simulink model "final_project"  (R2017b)
settings: Solver=FixedStepAuto  StartTime=0.0  StopTime=stopTime  FixedStep=stepSize  RelTol=1e-3
InitFcn:
  | final_project_init
values from neighbouring files (symbols this model uses):
  carrierFreq = 5e6    (= 5000000)    [final_project_init.m]
  dataRate = 10e6    (= 10000000)    [final_project_init.m]
  detection_threshold = 100    [final_project_init.m]
  mapper_LUT_I = [1 0.70710678 0.70710678 0 -0.70710678 0 -1 -0.70710678]    [final_project_init.m]
  mapper_LUT_Q = [0 0.70710678 -0.70710678 -1 0.70710678 1 0 -0.70710678]    [final_project_init.m]
  memSize = 1024    [final_project_init.m]
  pilot_size = length(pilot_bits)    [final_project_init.m]
  sampleRate = clockRate    (= 40000000)    [final_project_init.m]
  stepSize = 1/sampleRate    (= 2.5e-08)    [final_project_init.m]
  symbolRate = dataRate/3    (= 3333333.33333)    [final_project_init.m]
  wordLength = 12    [final_project_init.m]
undefined symbols (not defined in the file or in its folder): AdvDSPBChannelOutDisplay, AdvDSPBDMemDisplay, dpoly, dspba, dspba_ChannelInVis, dspba_ChannelOutVis, dspba_internal_get_channel_ports, dspba_internal_get_demux_ports, evalAionMaskParam, latency, primtype, UseDontCare, value
libraries: DSPBAPrim x252, DSPBAControl x44, DSPBABase x32, DSPBAFilters x12, DSPBAVectorUtil x4
(part 1 of 4)
settings Model: Creator=bennetp  LastModifiedBy=soren
settings SolverCC: AutoInsertRateTranBlk=on

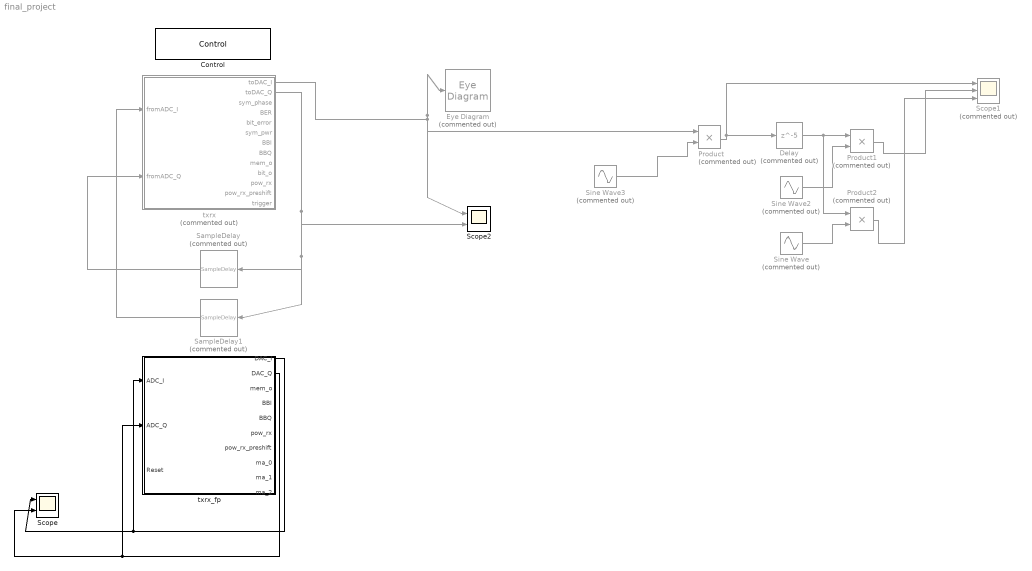
== system final_project ==
  Control : DSPBABase/Control  generate=off  language=VHDL  make_full_path=off  path_is_relative=on  autotestbench=on  signaldepth=2  coveragetestbench=off  logs=off  spacewidth=2  spacenum=1  addrwidth=10  datawidth=16  dataendian=Big Endian  hierarchicalnames=off  ramThresholdBits=-1  distRamThresholdBits=-1  mlabThresholdBits=-1  hardMultiplierThresholdLuts=-1  version=20150801  errorOnChanMismatch=1  errorOnGPIOMismatch=0  importModelsimResults=0  cycleAccurate=off  reinterpretCastMult=off  paramFile=final_project_params.xml
  Delay : Delay  Commented=on  DelayLength=5  InitialCondition=0  SampleTime=stepSize
  Eye Diagram : EyeDiagram  Commented=on
  Product : Product  Commented=on
  Product1 : Product  Commented=on
  Product2 : Product  Commented=on
  SampleDelay : DSPBAPrim/SampleDelay  Commented=on  primtype=sampdelay  nInputs=1  nOutputs=1  omode=Inherit via internal rule  otype=sfix(16)  scale=2^-15  rndmethod=Unbiased  factor=1  satmethod=Symmetric  shift_vec=[0 1 2 -1]  value=200  inPortNames=[' '; ' ';]  outPortNames=[' ']  dspbaimage=dspba_prim.jpg  text=dpoly(1, eye(1,value+1), 'z')  style=Optimised  visibilities=8 + 1024 + 2^17 + 2^18  flexible=off  slackgroup=0  augmented=0  version=20090407  advOptions=[]
  SampleDelay1 : DSPBAPrim/SampleDelay  Commented=on  primtype=sampdelay  nInputs=1  nOutputs=1  omode=Inherit via internal rule  otype=sfix(16)  scale=2^-15  rndmethod=Unbiased  factor=1  satmethod=Symmetric  shift_vec=[0 1 2 -1]  value=200  inPortNames=[' '; ' ';]  outPortNames=[' ']  dspbaimage=dspba_prim.jpg  text=dpoly(1, eye(1,value+1), 'z')  style=Optimised  visibilities=8 + 1024 + 2^17 + 2^18  flexible=off  slackgroup=0  augmented=0  version=20090407  advOptions=[]
  Scope : Scope  NumInputPorts=2
  Scope1 : Scope  Commented=on  NumInputPorts=3
  Scope2 : Scope  NumInputPorts=2
  Sine Wave : Sin  Commented=on  Frequency=carrierFreq*2*pi  Phase=pi  SampleTime=1/sampleRate
  Sine Wave2 : Sin  Commented=on  Frequency=carrierFreq*2*pi  Phase=pi/2  SampleTime=1/sampleRate
  Sine Wave3 : Sin  Commented=on  Frequency=carrierFreq*2*pi  Phase=pi/2  SampleTime=1/sampleRate
  txrx : Subsystem  Commented=on
  txrx_fp : Subsystem
  wires:
  Product1/1 -> Scope1/2
  Sine Wave2/1 -> Product1/2
  Product2/1 -> Scope1/3
  Sine Wave3/1 -> Product/2
  Delay/1 -> Product2/1, Product1/1
  txrx/2(toDAC_Q) -> SampleDelay1/1, SampleDelay/1, Scope2/2
  Product/1 -> Delay/1, Scope1/1
  Sine Wave/1 -> Product2/2
  txrx/1(toDAC_I) -> Eye Diagram/1, Product/1, Scope2/1
  SampleDelay/1 -> txrx/2(fromADC_Q)
  SampleDelay1/1 -> txrx/1(fromADC_I)
  txrx_fp/1(DAC_I) -> Scope/1, txrx_fp/1(ADC_I)
  txrx_fp/2(DAC_Q) -> Scope/2, txrx_fp/2(ADC_Q)

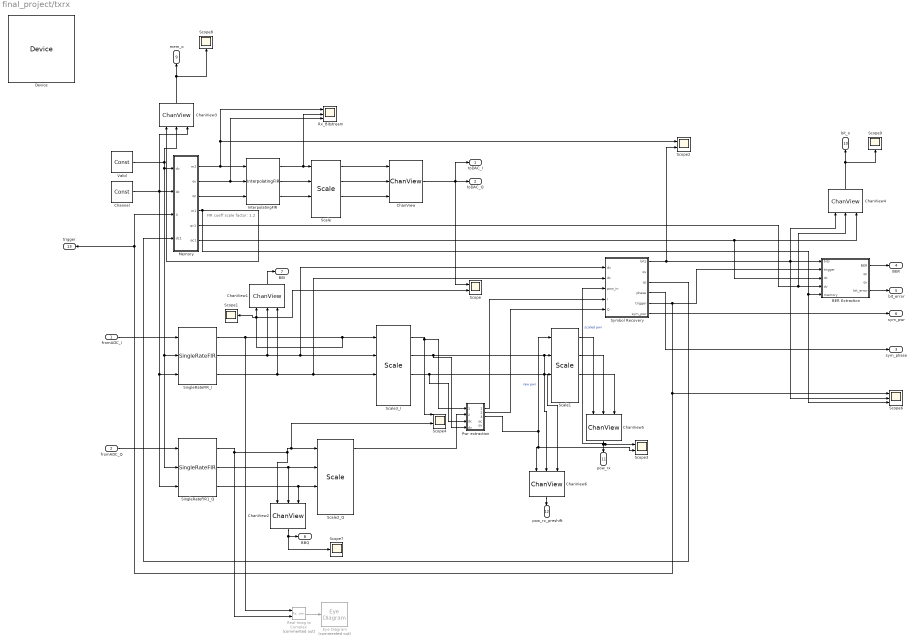
== system final_project/txrx ==
  note: FIR coeff scale factor: 1.2
  fromADC_I : Inport
  fromADC_Q : Inport  Port=2
  BER Extraction : Subsystem
  ChanView{,1..6} (7 alike) : DSPBABase/ChanView  nchans=1  chan_vector=[0]  outsvalid=off  latency=1  version=20090407
  Channel : DSPBAPrim/Const  primtype=const  nInputs=0  nOutputs=1  omode=Specify via dialog  otype=uint(8)  scale=1  rndmethod=Unbiased  factor=1  satmethod=Symmetric  shift_vec=[0 1 2 -1]  value=0  inPortNames=['+'; '+';]  outPortNames=[' ']  dspbaimage=dspba_prim.jpg  text=fprintf('%s', num2str(value));  style=Optimised  visibilities=8 + 1024  floatPrecision=float32_m23  version=20120820
  Device : DSPBABase/Device  family=Arria 10  stratix4device=Stratix IV E  hardcopy4device=HardCopy IV E  stratix5device=Stratix V GX  device=AUTO  speed=1  stratixSpeed=-5  stratix2Speed=-3  stratix3Speed=-2  stratix4gxSpeed=-2  stratix4gtSpeed=-1  cyclone2Speed=-6  cyclone3Speed=-7  arria2Speed=-4  cyclone4eSpeed=-8  stratix5Speed=-3  arria5Speed=-4  arriaSpeed=-6  cyclone3lsSpeed=-7  cyclone5Speed=-6  arria2gzSpeed=-3  nightFurySpeed=-2  ecp2Speed=-7  hardcopycompat=off  version=20140217  max10flashmode=off  max10nomeminit=off
  Eye Diagram : EyeDiagram  Commented=on
  InterpolatingFIR : DSPBAFilters/InterpolatingFIR  nInputRate=1  interp=sampleRate/dataRate  nchan=1  symmetry=Symmetrical  coef=fir.coeffs  addr=512  rwmode=Constant  nband=Use All Taps  exposebus=off  latency=8  version=20090407  recon=off  MM=[0,1,2,3,4,5,6,7,8,9,10,11,12,13,14,15]
  Memory : Subsystem
  Pwr extraction : Subsystem
  Real-Imag to Complex : RealImagToComplex  Commented=on
  Rx_Bitstream : Scope  NumInputPorts=3
  Scale : DSPBABase/Scale  otype=fixdt(1,12)  scale=1  rndmethod=Biased  factor=1  satmethod=Symmetric  shift_vec=13  latency=1  wideSimulation=off  version=20130807
  Scale1 : DSPBABase/Scale  otype=fixdt(1,wordLength)  scale=1  rndmethod=Biased  factor=1  satmethod=Symmetric  shift_vec=-11  latency=1  wideSimulation=off  version=20130807
  Scale2_Q : DSPBABase/Scale  otype=fixdt(1,wordLength)  scale=1  rndmethod=Biased  factor=1  satmethod=Symmetric  shift_vec=-3  latency=1  wideSimulation=off  version=20130807
  Scale3_I : DSPBABase/Scale  otype=fixdt(1,wordLength)  scale=1  rndmethod=Biased  factor=1  satmethod=Symmetric  shift_vec=-3  latency=1  wideSimulation=off  version=20130807
  Scope : Scope  NumInputPorts=2
  Scope{1,7..9} (4 alike) : Scope
  Scope2 : Scope  NumInputPorts=2
  Scope3 : Scope  NumInputPorts=2
  Scope4 : Scope  NumInputPorts=4
  Scope6 : Scope  NumInputPorts=3
  SingleRateFIR1_Q : DSPBAFilters/SingleRateFIR  nInputRate=40  nchan=1  symmetry=Symmetrical  coef=fir.coeffs  addr=512  rwmode=Read/Write  nband=Use All Taps  latency=4  exposebus=off  version=20090407  recon=off  MM=[0,1,2,3,4,5,6,7,8,9,10,11,12,13,14,15,16,17,18,19]
  SingleRateFIR_I : DSPBAFilters/SingleRateFIR  nInputRate=40  nchan=1  symmetry=Symmetrical  coef=fir.coeffs  addr=1024  rwmode=Read/Write  nband=Use All Taps  latency=4  exposebus=off  version=20090407  recon=off  MM=[0,1,2,3,4,5,6,7,8,9,10,11,12,13,14,15,16,17,18,19]
  Symbol Recovery : Subsystem
  Valid : DSPBAPrim/Const  primtype=const  nInputs=0  nOutputs=1  omode=boolean  otype=Boolean  scale=1  rndmethod=Unbiased  factor=1  satmethod=Symmetric  shift_vec=[0 1 2 -1]  value=1  inPortNames=['+'; '+';]  outPortNames=[' ']  dspbaimage=dspba_prim.jpg  text=fprintf('%s', num2str(value));  style=Optimised  visibilities=8 + 1024  floatPrecision=float32_m23  version=20120820
  toDAC_I : Outport
  toDAC_Q : Outport  Port=2
  sym_phase : Outport  Port=3
  BER : Outport  Port=4
  bit_error : Outport  Port=5
  sym_pwr : Outport  Port=6
  BBI : Outport  Port=7
  BBQ : Outport  Port=8
  mem_o : Outport  Port=9
  bit_o : Outport  Port=10
  pow_rx : Outport  Port=11
  pow_rx_preshift : Outport  Port=12
  trigger : Outport  Port=13
  wires:
  Valid/1 -> SingleRateFIR1_Q/2, SingleRateFIR_I/2, Memory/1(dv), ChanView3/2
  Channel/1 -> ChanView3/3, Memory/2(dc), SingleRateFIR1_Q/3, SingleRateFIR_I/3
  Memory/2(qv) -> Rx_Bitstream/3, InterpolatingFIR/2
  Memory/3(qc) -> InterpolatingFIR/3
  fromADC_I/1 -> SingleRateFIR_I/1
  fromADC_Q/1 -> SingleRateFIR1_Q/1
  Scale1/1 -> ChanView5/1
  Scale3_I/2 -> Pwr extraction/4(dv), ChanView6/2, Scale1/2
  Scale3_I/3 -> Pwr extraction/3(dc), ChanView6/3, Scale1/3
  ChanView/1 -> toDAC_I/1, toDAC_Q/1, Scope/1
  InterpolatingFIR/1 -> Rx_Bitstream/2, Scale/1
  InterpolatingFIR/2 -> Scale/2
  InterpolatingFIR/3 -> Scale/3
  Scale/1 -> ChanView/1
  Scale/2 -> ChanView/2
  Scale/3 -> ChanView/3
  Memory/1(m2) -> Scope2/1, Rx_Bitstream/1, InterpolatingFIR/1
  Symbol Recovery/1(bits) -> Scope2/2, BER Extraction/1(bits), ChanView4/1, Scope6/2
  Symbol Recovery/4(phase) -> sym_phase/1
  Memory/4(m1) -> ChanView3/1, Scope6/3, BER Extraction/5(memory)
  Memory/5(qv1) -> BER Extraction/4(dv), ChanView4/2
  Memory/6(qc1) -> BER Extraction/3(dc), ChanView4/3
  Symbol Recovery/5(trigger) -> Memory/3(trigger), trigger/1, Scope6/1, BER Extraction/2(trigger)
  Symbol Recovery/3(qc) -> Memory/4(dc1)
  BER Extraction/1(BER) -> BER/1
  BER Extraction/4(bit_error) -> bit_error/1
  Symbol Recovery/6(sym_pwr) -> sym_pwr/1
  SingleRateFIR1_Q/2 -> Scale2_Q/2, ChanView2/2
  SingleRateFIR1_Q/3 -> Scale2_Q/3, ChanView2/3
  SingleRateFIR_I/2 -> Scale3_I/2, Symbol Recovery/1(dv), ChanView1/2
  SingleRateFIR_I/3 -> Scale3_I/3, Symbol Recovery/2(dc), ChanView1/3
  Real-Imag to Complex/1 -> Eye Diagram/1
  ChanView2/1 -> Scope7/1, BBQ/1
  ChanView1/1 -> BBI/1
  ChanView3/1 -> mem_o/1, Scope8/1
  ChanView4/1 -> bit_o/1, Scope9/1
  Scale1/2 -> ChanView5/2
  Scale1/3 -> ChanView5/3
  ChanView5/1 -> pow_rx/1, Symbol Recovery/3(pow_in), Scope3/1  "scaled pwr"
  ChanView6/1 -> pow_rx_preshift/1
  SingleRateFIR1_Q/1 -> Scope4/3, Scale2_Q/1, ChanView2/1, Real-Imag to Complex/2
  SingleRateFIR_I/1 -> Scale3_I/1, Scope/2, Scope1/1, ChanView1/1, Real-Imag to Complex/1
  Pwr extraction/3(pwr) -> ChanView6/1, Scope3/2, Scale1/1  "raw pwr"
  Pwr extraction/1(Out1) -> Symbol Recovery/4(I)
  Pwr extraction/2(Out2) -> Symbol Recovery/5(Q)
  Scale2_Q/1 -> Pwr extraction/2(In2)
  Scale3_I/1 -> Pwr extraction/1(In1), Scope4/1

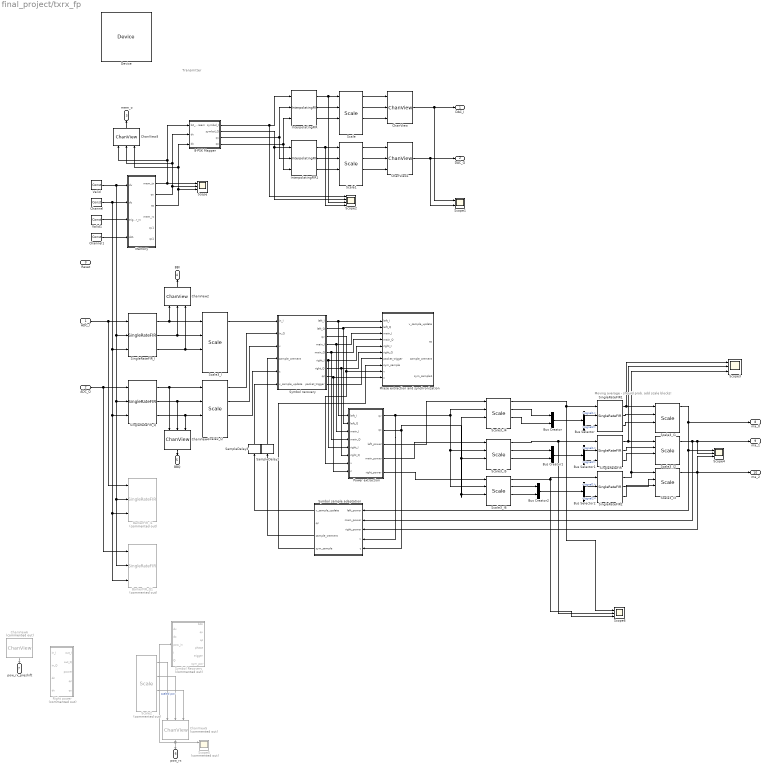
== system final_project/txrx_fp ==
  note: Moving average - should prob. add scale blocks!
  note: Transmitter
  ADC_I : Inport
  ADC_Q : Inport  Port=2
  Reset : Inport  Port=3
  8-PSK Mapper : Subsystem
  BarkerFIR_I1 : DSPBAFilters/SingleRateFIR  Commented=on  nInputRate=40  nchan=1  symmetry=Non Symmetrical  coef=barker_fir  addr=1024  rwmode=Read/Write  nband=Use All Taps  latency=2  exposebus=off  version=20090407  recon=off  MM=[0,1,2,3,4,5,6,7,8,9,10,11,12,13,14,15,16,17,18,19]
  BarkerFIR_Q1 : DSPBAFilters/SingleRateFIR  Commented=on  nInputRate=40  nchan=1  symmetry=Non Symmetrical  coef=barker_fir  addr=512  rwmode=Read/Write  nband=Use All Taps  latency=2  exposebus=off  version=20090407  recon=off  MM=[0,1,2,3,4,5,6,7,8,9,10,11,12,13,14,15,16,17,18,19]
  Bus Creator : BusCreator  Inputs=2
  Bus Creator1 : BusCreator  Inputs=2
  Bus Creator2 : BusCreator  Inputs=2
  Bus Selector : BusSelector  OutputSignals=signal1,signal2
  Bus Selector1 : BusSelector  OutputSignals=signal1,signal2
  Bus Selector2 : BusSelector  OutputSignals=signal1,signal2
  ChanView{,1..4} (5 alike) : DSPBABase/ChanView  nchans=1  chan_vector=[0]  outsvalid=off  latency=1  version=20090407
  ChanView5 : DSPBABase/ChanView  Commented=on  nchans=1  chan_vector=[0]  outsvalid=off  latency=1  version=20090407
  ChanView6 : DSPBABase/ChanView  Commented=on  nchans=1  chan_vector=[0]  outsvalid=off  latency=1  version=20090407
  Channel : DSPBAPrim/Const  primtype=const  nInputs=0  nOutputs=1  omode=Specify via dialog  otype=uint(8)  scale=1  rndmethod=Unbiased  factor=1  satmethod=Symmetric  shift_vec=[0 1 2 -1]  value=0  inPortNames=['+'; '+';]  outPortNames=[' ']  dspbaimage=dspba_prim.jpg  text=fprintf('%s', num2str(value));  style=Optimised  visibilities=8 + 1024  floatPrecision=float32_m23  version=20120820
  Channel1 : DSPBAPrim/Const  primtype=const  nInputs=0  nOutputs=1  omode=Specify via dialog  otype=uint(8)  scale=1  rndmethod=Unbiased  factor=1  satmethod=Symmetric  shift_vec=[0 1 2 -1]  value=0  inPortNames=['+'; '+';]  outPortNames=[' ']  dspbaimage=dspba_prim.jpg  text=fprintf('%s', num2str(value));  style=Optimised  visibilities=8 + 1024  floatPrecision=float32_m23  version=20120820
  Device : DSPBABase/Device  family=Arria 10  stratix4device=Stratix IV E  hardcopy4device=HardCopy IV E  stratix5device=Stratix V GX  device=AUTO  speed=1  stratixSpeed=-5  stratix2Speed=-3  stratix3Speed=-2  stratix4gxSpeed=-2  stratix4gtSpeed=-1  cyclone2Speed=-6  cyclone3Speed=-7  arria2Speed=-4  cyclone4eSpeed=-8  stratix5Speed=-3  arria5Speed=-4  arriaSpeed=-6  cyclone3lsSpeed=-7  cyclone5Speed=-6  arria2gzSpeed=-3  nightFurySpeed=-2  ecp2Speed=-7  hardcopycompat=off  version=20140217  max10flashmode=off  max10nomeminit=off
  InterpolatingFIR : DSPBAFilters/InterpolatingFIR  nInputRate=symbolRate/1e6  interp=3*sampleRate/dataRate  nchan=1  symmetry=Symmetrical  coef=fir.coeffs  addr=512  rwmode=Constant  nband=Use All Taps  exposebus=off  latency=8  version=20090407  recon=off  MM=[0,1,2,3,4,5,6,7,8,9,10,11,12,13,14,15]
  InterpolatingFIR1 : DSPBAFilters/InterpolatingFIR  nInputRate=symbolRate/1e6  interp=3*sampleRate/dataRate  nchan=1  symmetry=Symmetrical  coef=fir.coeffs  addr=512  rwmode=Constant  nband=Use All Taps  exposebus=off  latency=8  version=20090407  recon=off  MM=[0,1,2,3,4,5,6,7,8,9,10,11,12,13,14,15]
  Memory : Subsystem
  Phase extraction and synchronization : Subsystem
  Power extraction : Subsystem
  Right power : Subsystem  Commented=on
  SampleDelay1 : DSPBAPrim/SampleDelay  primtype=sampdelay  nInputs=1  nOutputs=1  omode=Inherit via internal rule  otype=sfix(16)  scale=2^-15  rndmethod=Unbiased  factor=1  satmethod=Symmetric  shift_vec=[0 1 2 -1]  value=1  inPortNames=[' '; ' ';]  outPortNames=[' ']  dspbaimage=dspba_prim.jpg  text=dpoly(1, eye(1,value+1), 'z')  style=Optimised  visibilities=8 + 1024 + 2^17 + 2^18  flexible=off  slackgroup=0  augmented=0  version=20090407  advOptions=[]
  SampleDelay3 : DSPBAPrim/SampleDelay  primtype=sampdelay  nInputs=1  nOutputs=1  omode=Inherit via internal rule  otype=sfix(16)  scale=2^-15  rndmethod=Unbiased  factor=1  satmethod=Symmetric  shift_vec=[0 1 2 -1]  value=1  inPortNames=[' '; ' ';]  outPortNames=[' ']  dspbaimage=dspba_prim.jpg  text=dpoly(1, eye(1,value+1), 'z')  style=Optimised  visibilities=8 + 1024 + 2^17 + 2^18  flexible=off  slackgroup=0  augmented=0  version=20090407  advOptions=[]
  Scale : DSPBABase/Scale  otype=fixdt(1,12)  scale=1  rndmethod=Biased  factor=1  satmethod=Symmetric  shift_vec=1  latency=1  wideSimulation=off  version=20130807
  Scale1 : DSPBABase/Scale  otype=fixdt(1,12)  scale=1  rndmethod=Biased  factor=1  satmethod=Symmetric  shift_vec=1  latency=1  wideSimulation=off  version=20130807
  Scale2 : DSPBABase/Scale  Commented=on  otype=fixdt(1,wordLength)  scale=1  rndmethod=Biased  factor=1  satmethod=Symmetric  shift_vec=-11  latency=1  wideSimulation=off  version=20130807
  Scale2_Q : DSPBABase/Scale  otype=fixdt(1,wordLength)  scale=1  rndmethod=Biased  factor=1  satmethod=Symmetric  shift_vec=-2  latency=1  wideSimulation=off  version=20130807
  Scale3_I : DSPBABase/Scale  otype=fixdt(1,wordLength)  scale=1  rndmethod=Biased  factor=1  satmethod=Symmetric  shift_vec=-2  latency=1  wideSimulation=off  version=20130807
  Scale3_I1 : DSPBABase/Scale  otype=fixdt(1,wordLength)  scale=1  rndmethod=Biased  factor=1  satmethod=Symmetric  shift_vec=-3  latency=1  wideSimulation=off  version=20130807
  Scale3_I2 : DSPBABase/Scale  otype=fixdt(1,wordLength)  scale=1  rndmethod=Biased  factor=1  satmethod=Symmetric  shift_vec=-3  latency=1  wideSimulation=off  version=20130807
  Scale3_I3 : DSPBABase/Scale  otype=fixdt(1,wordLength)  scale=1  rndmethod=Biased  factor=1  satmethod=Symmetric  shift_vec=-3  latency=1  wideSimulation=off  version=20130807
  Scale3_I4 : DSPBABase/Scale  otype=fixdt(1,18)  scale=1  rndmethod=Biased  factor=1  satmethod=Symmetric  shift_vec=-7  latency=1  wideSimulation=off  version=20130807
  Scale3_I5 : DSPBABase/Scale  otype=fixdt(1,18)  scale=1  rndmethod=Biased  factor=1  satmethod=Symmetric  shift_vec=-7  latency=1  wideSimulation=off  version=20130807
  Scale3_I6 : DSPBABase/Scale  otype=fixdt(1,18)  scale=1  rndmethod=Biased  factor=1  satmethod=Symmetric  shift_vec=-7  latency=1  wideSimulation=off  version=20130807
  Scope{,3..4,6} (4 alike) : Scope  NumInputPorts=3
  Scope1 : Scope  NumInputPorts=2
  Scope2 : Scope  NumInputPorts=4
  Scope5 : Scope  Commented=on  NumInputPorts=2
  SingleRateFIR : DSPBAFilters/SingleRateFIR  nInputRate=40  nchan=1  symmetry=Symmetrical  coef=moving_avg_fir  addr=2048  rwmode=Constant  nband=Use All Taps  latency=2  exposebus=off  version=20090407  recon=off  MM=[0,1,2,3,4,5,6,7,8,9,10,11,12,13,14,15,16,17,18,19]
  SingleRateFIR1 : DSPBAFilters/SingleRateFIR  nInputRate=40  nchan=1  symmetry=Symmetrical  coef=moving_avg_fir  addr=2048  rwmode=Constant  nband=Use All Taps  latency=2  exposebus=off  version=20090407  recon=off  MM=[0,1,2,3,4,5,6,7,8,9,10,11,12,13,14,15,16,17,18,19]
  SingleRateFIR2 : DSPBAFilters/SingleRateFIR  nInputRate=40  nchan=1  symmetry=Symmetrical  coef=moving_avg_fir  addr=2048  rwmode=Constant  nband=Use All Taps  latency=2  exposebus=off  version=20090407  recon=off  MM=[0,1,2,3,4,5,6,7,8,9,10,11,12,13,14,15,16,17,18,19]
  SingleRateFIR_I : DSPBAFilters/SingleRateFIR  nInputRate=40  nchan=1  symmetry=Symmetrical  coef=fir.coeffs  addr=1024  rwmode=Read/Write  nband=Use All Taps  latency=2  exposebus=off  version=20090407  recon=off  MM=[0,1,2,3,4,5,6,7,8,9,10,11,12,13,14,15,16,17,18,19]
  SingleRateFIR_Q : DSPBAFilters/SingleRateFIR  nInputRate=40  nchan=1  symmetry=Symmetrical  coef=fir.coeffs  addr=512  rwmode=Read/Write  nband=Use All Taps  latency=2  exposebus=off  version=20090407  recon=off  MM=[0,1,2,3,4,5,6,7,8,9,10,11,12,13,14,15,16,17,18,19]
  Symbol Recovery : Subsystem  Commented=on
  Symbol recovery : Subsystem
  Symbol sample adaptation : Subsystem
  Valid : DSPBAPrim/Const  primtype=const  nInputs=0  nOutputs=1  omode=boolean  otype=Boolean  scale=1  rndmethod=Unbiased  factor=1  satmethod=Symmetric  shift_vec=[0 1 2 -1]  value=1  inPortNames=['+'; '+';]  outPortNames=[' ']  dspbaimage=dspba_prim.jpg  text=fprintf('%s', num2str(value));  style=Optimised  visibilities=8 + 1024  floatPrecision=float32_m23  version=20120820
  Valid1 : DSPBAPrim/Const  primtype=const  nInputs=0  nOutputs=1  omode=boolean  otype=Boolean  scale=1  rndmethod=Unbiased  factor=1  satmethod=Symmetric  shift_vec=[0 1 2 -1]  value=0  inPortNames=['+'; '+';]  outPortNames=[' ']  dspbaimage=dspba_prim.jpg  text=fprintf('%s', num2str(value));  style=Optimised  visibilities=8 + 1024  floatPrecision=float32_m23  version=20120820
  DAC_I : Outport
  DAC_Q : Outport  Port=2
  mem_o : Outport  Port=3
  BBI : Outport  Port=4
  BBQ : Outport  Port=5
  pow_rx : Outport  Port=6
  pow_rx_preshift : Outport  Port=7
  ma_0 : Outport  Port=8
  ma_1 : Outport  Port=9
  ma_2 : Outport  Port=10
  wires:
  Valid/1 -> Memory/1(dv), SingleRateFIR_I/2, BarkerFIR_Q1/2, BarkerFIR_I1/2, SingleRateFIR_Q/2
  Channel/1 -> Memory/2(dc), SingleRateFIR_I/3, BarkerFIR_Q1/3, BarkerFIR_I1/3, SingleRateFIR_Q/3
  Memory/1(mem_tx) -> ChanView3/1, 8-PSK Mapper/1(bit_stream), Scope/1
  8-PSK Mapper/1(symbol_I) -> InterpolatingFIR/1, Scope2/1
  8-PSK Mapper/2(symbol_Q) -> Scope2/2, InterpolatingFIR1/1
  ChanView3/1 -> mem_o/1
  Memory/2(qv) -> ChanView3/2, 8-PSK Mapper/2(dv), Scope/2
  Memory/3(qc) -> ChanView3/3, 8-PSK Mapper/3(dc), Scope/3
  InterpolatingFIR/1 -> Scale/1, Scope2/3
  InterpolatingFIR1/1 -> Scope2/4, Scale1/1
  Scale/1 -> ChanView/1
  Scale1/1 -> ChanView1/1
  InterpolatingFIR1/2 -> Scale1/2
  InterpolatingFIR1/3 -> Scale1/3
  Scale1/3 -> ChanView1/3
  Scale1/2 -> ChanView1/2
  Scale/2 -> ChanView/2
  Scale/3 -> ChanView/3
  InterpolatingFIR/2 -> Scale/2
  InterpolatingFIR/3 -> Scale/3
  ChanView/1 -> DAC_I/1, Scope1/1
  ChanView1/1 -> DAC_Q/1, Scope1/2
  8-PSK Mapper/3(qv) -> InterpolatingFIR/2, InterpolatingFIR1/2
  8-PSK Mapper/4(qc) -> InterpolatingFIR1/3, InterpolatingFIR/3
  ChanView5/1 -> Scope5/1, Symbol Recovery/3(pow_in), pow_rx/1  "scaled pwr"
  Scale2/2 -> ChanView5/2
  ChanView2/1 -> BBI/1
  Scale2/1 -> ChanView5/1
  Scale2/3 -> ChanView5/3
  ChanView4/1 -> BBQ/1
  ChanView6/1 -> pow_rx_preshift/1
  ADC_I/1 -> BarkerFIR_I1/1, SingleRateFIR_I/1
  ADC_Q/1 -> BarkerFIR_Q1/1, SingleRateFIR_Q/1
  SingleRateFIR_I/1 -> ChanView2/1, Scale3_I/1
  SingleRateFIR_I/2 -> Scale3_I/2, ChanView2/2
  SingleRateFIR_I/3 -> Scale3_I/3, ChanView2/3
  SingleRateFIR_Q/3 -> Scale2_Q/3, ChanView4/3
  SingleRateFIR_Q/2 -> Scale2_Q/2, ChanView4/2
  SingleRateFIR_Q/1 -> Scale2_Q/1, ChanView4/1
  Scale3_I/1 -> Symbol recovery/1(in_I)
  Scale2_Q/1 -> Symbol recovery/2(in_Q)
  Scale2_Q/2 -> Symbol recovery/3(v)
  Scale2_Q/3 -> Symbol recovery/5(c)
  Symbol recovery/1(left_I) -> Power extraction/1(left_I), Phase extraction and synchronization/1(left_I)
  Symbol recovery/2(left_Q) -> Power extraction/2(left_Q), Phase extraction and synchronization/2(left_Q)
  Symbol recovery/3(qv) -> Power extraction/7(v), Phase extraction and synchronization/9(v)
  Symbol recovery/4(main_I) -> Power extraction/3(main_I), Phase extraction and synchronization/3(main_I)
  Symbol recovery/5(main_Q) -> Phase extraction and synchronization/4(main_Q), Power extraction/4(main_Q)
  Symbol recovery/7(right_Q) -> Power extraction/6(right_Q), Phase extraction and synchronization/6(right_Q)
  Symbol recovery/8(qc) -> Power extraction/8(c), Phase extraction and synchronization/10(c)
  Symbol sample adaptation/3(sample_crement) -> SampleDelay1/1
  Power extraction/2(qc) -> Symbol sample adaptation/5(c), Scale3_I5/3, Scale3_I4/3, Scale3_I6/3
  Power extraction/1(qv) -> Symbol sample adaptation/4(v), Scale3_I6/2, Scale3_I5/2, Scale3_I4/2
  SingleRateFIR1/1 -> Scale3_I1/1, Scope3/1
  SingleRateFIR/1 -> Scale3_I2/1, Scope3/2
  SingleRateFIR2/1 -> Scale3_I3/1, Scope3/3
  Symbol sample adaptation/1(v_sample_update) -> SampleDelay3/1
  SampleDelay3/1 -> Symbol recovery/6(v_sample_update)
  SampleDelay1/1 -> Symbol recovery/4(sample_crement)
  Symbol recovery/9(packet_trigger) -> Phase extraction and synchronization/7(packet_trigger)
  Symbol sample adaptation/4(sym_sample) -> Phase extraction and synchronization/8(sym_sample)
  Symbol recovery/6(right_I) -> Phase extraction and synchronization/5(right_I), Power extraction/5(right_I)
  SingleRateFIR1/2 -> Scale3_I1/2
  SingleRateFIR1/3 -> Scale3_I1/3
  SingleRateFIR/2 -> Scale3_I2/2
  SingleRateFIR/3 -> Scale3_I2/3
  SingleRateFIR2/2 -> Scale3_I3/2
  SingleRateFIR2/3 -> Scale3_I3/3
  Scale3_I1/1 -> ma_0/1, Symbol sample adaptation/1(left_power), Scope4/1
  Scale3_I2/1 -> Symbol sample adaptation/2(main_power), ma_1/1, Scope4/2
  Channel1/1 -> Memory/4(dc1)
  Valid1/1 -> Memory/3(trigger_rx)
  Scale3_I3/1 -> ma_2/1, Symbol sample adaptation/3(right_power), Scope4/3
  Power extraction/3(left_power) -> Scale3_I4/1
  Power extraction/4(main_power) -> Scale3_I5/1
  Power extraction/5(right_power) -> Scale3_I6/1
  Scale3_I4/1 -> Scope6/1, SingleRateFIR1/1
  Scale3_I5/1 -> Scope6/2, SingleRateFIR/1
  Scale3_I6/1 -> SingleRateFIR2/1, Scope6/3
  Scale3_I4/2 -> Bus Creator/1
  Scale3_I4/3 -> Bus Creator/2
  Scale3_I5/2 -> Bus Creator1/1
  Scale3_I5/3 -> Bus Creator1/2
  Scale3_I6/2 -> Bus Creator2/1
  Scale3_I6/3 -> Bus Creator2/2
  Bus Creator/1 -> Bus Selector/1
  Bus Selector/1 -> SingleRateFIR1/2  "<signal1>"
  Bus Selector/2 -> SingleRateFIR1/3  "<signal2>"
  Bus Selector1/1 -> SingleRateFIR/2  "<signal1>"
  Bus Selector1/2 -> SingleRateFIR/3  "<signal2>"
  Bus Selector2/1 -> SingleRateFIR2/2  "<signal1>"
  Bus Selector2/2 -> SingleRateFIR2/3  "<signal2>"
  Bus Creator1/1 -> Bus Selector1/1
  Bus Creator2/1 -> Bus Selector2/1

== system final_project/txrx/BER Extraction ==
  note: BER Computation
  bits : Inport
  trigger : Inport  Port=2
  dc : Inport  Port=3
  dv : Inport  Port=4
  memory : Inport  Port=5
  And : DSPBAPrim/And  primtype=and  nInputs=2  nOutputs=1  omode=Inherit via internal rule  otype=sfix(16)  scale=2^-15  rndmethod=Unbiased  factor=1  satmethod=Symmetric  shift_vec=[0 1 2 -1]  value=0  inPortNames=[' '; ' '; ' '; ' '; ' '; ' '; ' '; ' '; ' '; ' '; ' '; ' '; ' '; ' '; ' '; ' '; ]  outPortNames=[' ']  dspbaimage=dspba_prim.jpg  text=fprintf('&');  style=Optimised  visibilities=8+2  version=20090407
  Bit counter : DSPBAPrim/Counter  Commented=on  primtype=counter  nInputs=1  nOutputs=1  omode=Inherit via internal rule  otype=ufix(16)  scale=2^-0  rndmethod=Unbiased  factor=1  satmethod=Symmetric  shift_vec=[0 1 2 -1]  value=[0 memSize 1]  inPortNames=[' '; ' ';]  outPortNames=[' ']  dspbaimage=dspba_prim.jpg  text=fprintf('counter\n[%d %d %d]', value(1), value(2), value(3));  style=Optimised  visibilities=8 + 1024  version=20090407
  ChannelIn : DSPBAPrim/ChannelIn  primtype=channelin  nInputs=dspba_internal_get_channel_ports(gcb)  nOutputs=dspba_internal_get_channel_ports(gcb)  omode=Inherit via internal rule  otype=sfix(16)  scale=2^-15  rndmethod=Unbiased  factor=1  satmethod=Symmetric  shift_vec=[0 1 2 -1]  value=3  inPortNames=['v'; 'c'; '0'; '1'; '2'; '3'; '4'; '5'; '6'; '7'; '8'; '9'; 'A'; 'B'; 'D'; 'E'; 'F'; 'G'; 'H'; 'I'; 'J'; 'K'; 'L'; 'M'; 'N'; 'O'; 'P'; 'Q'; 'R'; 'S'; 'T'; 'U'; 'W'; 'X'; 'Y'; 'Z']  outPortNames=['v'; 'c'; '0'; '1'; '2'; '3'; '4'; '5'; '6'; '7'; '8'; '9'; 'A'; 'B'; 'D'; 'E'; 'F'; 'G'; 'H'; 'I'; 'J'; 'K'; 'L'; 'M'; 'N'; 'O'; 'P'; 'Q'; 'R'; 'S'; 'T'; 'U'; 'W'; 'X'; 'Y'; 'Z']  dspbaimage=dspba_prim.jpg  text=fprintf('In');  style=Optimised  dataSignals=3  foldingEnabled=off  channels=1  sampleRate=200  packetBeginPresent=off  packetBeginEnabled=off  visibilities=dspba_ChannelInVis(gcb)  latencyCorrection=0  scheduleOrigin=on  version=20141013
  ChannelOut : DSPBAPrim/ChannelOut  primtype=channelout  nInputs=dspba_internal_get_channel_ports(gcb)  nOutputs=dspba_internal_get_channel_ports(gcb)  omode=Inherit via internal rule  otype=sfix(16)  scale=2^-15  rndmethod=Unbiased  factor=1  satmethod=Symmetric  shift_vec=[0 1 2 -1]  value=2  inPortNames=['v'; 'c'; '0'; '1'; '2'; '3'; '4'; '5'; '6'; '7'; '8'; '9'; 'A'; 'B'; 'D'; 'E'; 'F'; 'G'; 'H'; 'I'; 'J'; 'K'; 'L'; 'M'; 'N'; 'O'; 'P'; 'Q'; 'R'; 'S'; 'T'; 'U'; 'W'; 'X'; 'Y'; 'Z']  outPortNames=['v'; 'c'; '0'; '1'; '2'; '3'; '4'; '5'; '6'; '7'; '8'; '9'; 'A'; 'B'; 'D'; 'E'; 'F'; 'G'; 'H'; 'I'; 'J'; 'K'; 'L'; 'M'; 'N'; 'O'; 'P'; 'Q'; 'R'; 'S'; 'T'; 'U'; 'W'; 'X'; 'Y'; 'Z']  dspbaimage=dspba_prim.jpg  text=fprintf('Out%s', AdvDSPBChannelOutDisplay(latency));  style=Optimised  dataSignals=2  foldingEnabled=off  channels=1  sampleRate=200  packetBeginPresent=off  packetBeginEnabled=off  visibilities=dspba_ChannelOutVis(gcb)  latency=0  latencyCorrection=0  version=20141013
  CmpEQ : DSPBAPrim/CmpEQ  Commented=on  primtype=cmpeq  nInputs=2  nOutputs=1  omode=boolean  otype=sfix(16)  scale=2^-15  rndmethod=Unbiased  factor=1  satmethod=Symmetric  shift_vec=[0 1 2 -1]  value=0  inPortNames=[' '; ' ';]  outPortNames=[' ']  dspbaimage=dspba_prim.jpg  text=fprintf('==');  style=Optimised  visibilities=0  advOptions=[]  version=20130117
  CmpNE : DSPBAPrim/CmpNE  primtype=cmpne  nInputs=2  nOutputs=1  omode=boolean  otype=sfix(16)  scale=2^-15  rndmethod=Unbiased  factor=1  satmethod=Symmetric  shift_vec=[0 1 2 -1]  value=0  inPortNames=[' '; ' ';]  outPortNames=[' ']  dspbaimage=dspba_prim.jpg  text=fprintf('~=');  style=Optimised  visibilities=0  advOptions=[]  version=20130117
  Const : DSPBAPrim/Const  Commented=on  primtype=const  nInputs=0  nOutputs=1  omode=Inherit via internal rule  otype=sfix(16)  scale=2^-15  rndmethod=Unbiased  factor=1  satmethod=Symmetric  shift_vec=[0 1 2 -1]  value=0  inPortNames=['+'; '+';]  outPortNames=[' ']  dspbaimage=dspba_prim.jpg  text=fprintf('%s', num2str(value));  style=Optimised  visibilities=8 + 1024  floatPrecision=float32_m23  version=20120820
  Const1 : DSPBAPrim/Const  primtype=const  nInputs=0  nOutputs=1  omode=Inherit via internal rule  otype=sfix(16)  scale=2^-15  rndmethod=Unbiased  factor=1  satmethod=Symmetric  shift_vec=[0 1 2 -1]  value=0  inPortNames=['+'; '+';]  outPortNames=[' ']  dspbaimage=dspba_prim.jpg  text=fprintf('%s', num2str(value));  style=Optimised  visibilities=8 + 1024  floatPrecision=float32_m23  version=20120820
  Divide : DSPBAPrim/Divide  Commented=on  primtype=divide  nInputs=2  nOutputs=1  omode=Inherit via internal rule  otype=sfix(16)  scale=2^-15  rndmethod=Unbiased  factor=1  satmethod=Symmetric  shift_vec=[0 1 2 -1]  value=round([0:255]/17)  inPortNames=[' '; ' ';]  outPortNames=[' ']  dspbaimage=dspba_prim.jpg  text=fprintf('a\n----\nb');  style=Optimised  visibilities=8+2^17+2^18  floatRounding=correct  advOptions=[]  version=20130115
  Error counter : DSPBAPrim/Counter  Commented=on  primtype=counter  nInputs=1  nOutputs=1  omode=Inherit via internal rule  otype=ufix(16)  scale=2^-0  rndmethod=Unbiased  factor=1  satmethod=Symmetric  shift_vec=[0 1 2 -1]  value=[0 memSize 1]  inPortNames=[' '; ' ';]  outPortNames=[' ']  dspbaimage=dspba_prim.jpg  text=fprintf('counter\n[%d %d %d]', value(1), value(2), value(3));  style=Optimised  visibilities=8 + 1024  version=20090407
  Or : DSPBAPrim/Or  Commented=on  primtype=or  nInputs=2  nOutputs=1  omode=Inherit via internal rule  otype=sfix(16)  scale=2^-15  rndmethod=Unbiased  factor=1  satmethod=Symmetric  shift_vec=[0 1 2 -1]  value=0  inPortNames=[' '; ' '; ' '; ' '; ' '; ' '; ' '; ' '; ' '; ' '; ' '; ' '; ' '; ' '; ' '; ' '; ]  outPortNames=[' ']  dspbaimage=dspba_prim.jpg  text=fprintf('|');  style=Optimised  visibilities=8+2  version=20090407
  Scope : Scope  NumInputPorts=4
  SynthesisInfo : DSPBAPrim/SynthesisInfo  primtype=synthinfo  nInputs=0  nOutputs=0  omode=Inherit via internal rule  otype=sfix(16)  scale=2^-15  rndmethod=Truncate  factor=1  satmethod=Symmetric  shift_vec=[0 1 2 -1]  value=99  inPortNames=[' '; ' ';]  outPortNames=[' ']  dspbaimage=dspba_prim_ctrl.jpg  text=fprintf('Style=%s', style);  style=Scheduled  visibilities=2^17+2^18+2^19+2^20  constraintInUse=off  constraintRelation=>  constraintLimit=2  bitAccurate=off  version=20150220
  mem loop compensate : DSPBAPrim/SampleDelay  primtype=sampdelay  nInputs=1  nOutputs=1  omode=Inherit via internal rule  otype=sfix(16)  scale=2^-15  rndmethod=Unbiased  factor=1  satmethod=Symmetric  shift_vec=[0 1 2 -1]  value=5  inPortNames=[' '; ' ';]  outPortNames=[' ']  dspbaimage=dspba_prim.jpg  text=dpoly(1, eye(1,value+1), 'z')  style=Optimised  visibilities=8 + 1024 + 2^17 + 2^18  flexible=off  slackgroup=0  augmented=0  version=20090407  advOptions=[]
  BER : Outport
  qc : Outport  Port=2
  qv : Outport  Port=3
  bit_error : Outport  Port=4
  wires:
  ChannelOut/3 -> BER/1
  bits/1 -> ChannelIn/3
  trigger/1 -> ChannelIn/4
  dc/1 -> ChannelIn/2
  dv/1 -> ChannelIn/1
  memory/1 -> ChannelIn/5
  ChannelIn/3 -> mem loop compensate/1
  ChannelIn/1 -> Bit counter/1, ChannelOut/1
  ChannelIn/2 -> ChannelOut/2
  ChannelOut/1 -> qv/1
  ChannelOut/2 -> qc/1
  ChannelIn/5 -> Scope/3, CmpNE/2
  CmpNE/1 -> And/1
  ChannelIn/4 -> And/2
  And/1 -> ChannelOut/4, Scope/1, Error counter/1
  mem loop compensate/1 -> CmpNE/1, Scope/2
  Error counter/1 -> Divide/1
  Bit counter/1 -> Or/1, CmpEQ/1
  Const/1 -> CmpEQ/2
  CmpEQ/1 -> Or/2
  Or/1 -> Divide/2
  Divide/1 -> Scope/4
  ChannelOut/4 -> bit_error/1
  Const1/1 -> ChannelOut/3

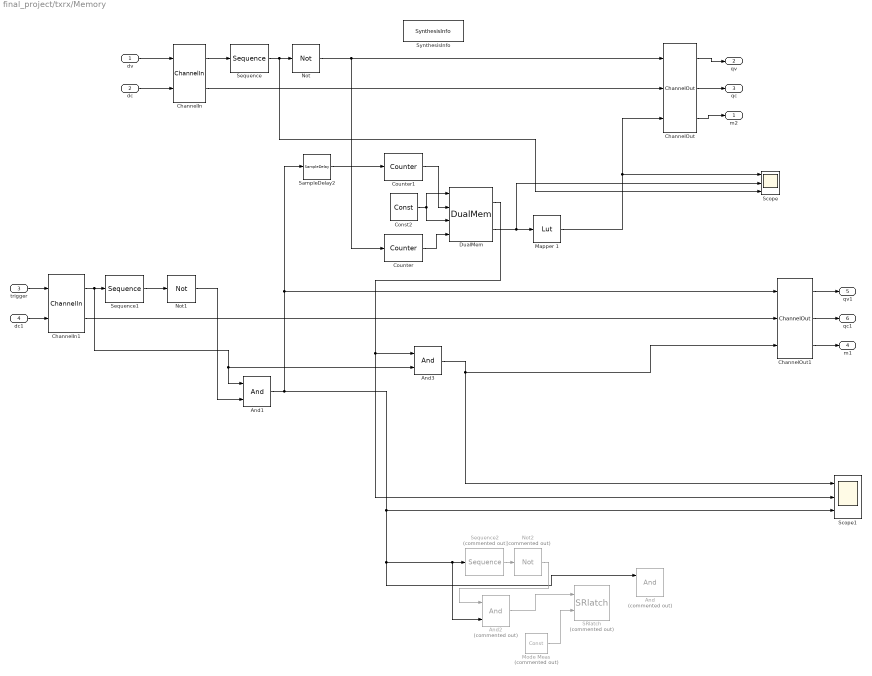
== system final_project/txrx/Memory ==
  dv : Inport
  dc : Inport  Port=2
  trigger : Inport  Port=3
  dc1 : Inport  Port=4
  And : DSPBAPrim/And  Commented=on  primtype=and  nInputs=2  nOutputs=1  omode=Inherit via internal rule  otype=sfix(16)  scale=2^-15  rndmethod=Unbiased  factor=1  satmethod=Symmetric  shift_vec=[0 1 2 -1]  value=0  inPortNames=[' '; ' '; ' '; ' '; ' '; ' '; ' '; ' '; ' '; ' '; ' '; ' '; ' '; ' '; ' '; ' '; ]  outPortNames=[' ']  dspbaimage=dspba_prim.jpg  text=fprintf('&');  style=Optimised  visibilities=8+2  version=20090407
  And1 : DSPBAPrim/And  primtype=and  nInputs=2  nOutputs=1  omode=Inherit via internal rule  otype=sfix(16)  scale=2^-15  rndmethod=Unbiased  factor=1  satmethod=Symmetric  shift_vec=[0 1 2 -1]  value=0  inPortNames=[' '; ' '; ' '; ' '; ' '; ' '; ' '; ' '; ' '; ' '; ' '; ' '; ' '; ' '; ' '; ' '; ]  outPortNames=[' ']  dspbaimage=dspba_prim.jpg  text=fprintf('&');  style=Optimised  visibilities=8+2  version=20090407
  And2 : DSPBAPrim/And  Commented=on  primtype=and  nInputs=2  nOutputs=1  omode=Inherit via internal rule  otype=sfix(16)  scale=2^-15  rndmethod=Unbiased  factor=1  satmethod=Symmetric  shift_vec=[0 1 2 -1]  value=0  inPortNames=[' '; ' '; ' '; ' '; ' '; ' '; ' '; ' '; ' '; ' '; ' '; ' '; ' '; ' '; ' '; ' '; ]  outPortNames=[' ']  dspbaimage=dspba_prim.jpg  text=fprintf('&');  style=Optimised  visibilities=8+2  version=20090407
  And3 : DSPBAPrim/And  primtype=and  nInputs=2  nOutputs=1  omode=Inherit via internal rule  otype=sfix(16)  scale=2^-15  rndmethod=Unbiased  factor=1  satmethod=Symmetric  shift_vec=[0 1 2 -1]  value=0  inPortNames=[' '; ' '; ' '; ' '; ' '; ' '; ' '; ' '; ' '; ' '; ' '; ' '; ' '; ' '; ' '; ' '; ]  outPortNames=[' ']  dspbaimage=dspba_prim.jpg  text=fprintf('&');  style=Optimised  visibilities=8+2  version=20090407
  ChannelIn : DSPBAPrim/ChannelIn  primtype=channelin  nInputs=dspba_internal_get_channel_ports(gcb)  nOutputs=dspba_internal_get_channel_ports(gcb)  omode=Inherit via internal rule  otype=sfix(16)  scale=2^-15  rndmethod=Unbiased  factor=1  satmethod=Symmetric  shift_vec=[0 1 2 -1]  value=0  inPortNames=['v'; 'c'; '0'; '1'; '2'; '3'; '4'; '5'; '6'; '7'; '8'; '9'; 'A'; 'B'; 'D'; 'E'; 'F'; 'G'; 'H'; 'I'; 'J'; 'K'; 'L'; 'M'; 'N'; 'O'; 'P'; 'Q'; 'R'; 'S'; 'T'; 'U'; 'W'; 'X'; 'Y'; 'Z']  outPortNames=['v'; 'c'; '0'; '1'; '2'; '3'; '4'; '5'; '6'; '7'; '8'; '9'; 'A'; 'B'; 'D'; 'E'; 'F'; 'G'; 'H'; 'I'; 'J'; 'K'; 'L'; 'M'; 'N'; 'O'; 'P'; 'Q'; 'R'; 'S'; 'T'; 'U'; 'W'; 'X'; 'Y'; 'Z']  dspbaimage=dspba_prim.jpg  text=fprintf('In');  style=Optimised  dataSignals=0  foldingEnabled=off  channels=1  sampleRate=200  packetBeginPresent=off  packetBeginEnabled=off  visibilities=dspba_ChannelInVis(gcb)  latencyCorrection=0  scheduleOrigin=on  version=20141013
  ChannelIn1 : DSPBAPrim/ChannelIn  primtype=channelin  nInputs=dspba_internal_get_channel_ports(gcb)  nOutputs=dspba_internal_get_channel_ports(gcb)  omode=Inherit via internal rule  otype=sfix(16)  scale=2^-15  rndmethod=Unbiased  factor=1  satmethod=Symmetric  shift_vec=[0 1 2 -1]  value=0  inPortNames=['v'; 'c'; '0'; '1'; '2'; '3'; '4'; '5'; '6'; '7'; '8'; '9'; 'A'; 'B'; 'D'; 'E'; 'F'; 'G'; 'H'; 'I'; 'J'; 'K'; 'L'; 'M'; 'N'; 'O'; 'P'; 'Q'; 'R'; 'S'; 'T'; 'U'; 'W'; 'X'; 'Y'; 'Z']  outPortNames=['v'; 'c'; '0'; '1'; '2'; '3'; '4'; '5'; '6'; '7'; '8'; '9'; 'A'; 'B'; 'D'; 'E'; 'F'; 'G'; 'H'; 'I'; 'J'; 'K'; 'L'; 'M'; 'N'; 'O'; 'P'; 'Q'; 'R'; 'S'; 'T'; 'U'; 'W'; 'X'; 'Y'; 'Z']  dspbaimage=dspba_prim.jpg  text=fprintf('In');  style=Optimised  dataSignals=0  foldingEnabled=off  channels=1  sampleRate=200  packetBeginPresent=off  packetBeginEnabled=off  visibilities=dspba_ChannelInVis(gcb)  latencyCorrection=0  scheduleOrigin=on  version=20141013
  ChannelOut : DSPBAPrim/ChannelOut  primtype=channelout  nInputs=dspba_internal_get_channel_ports(gcb)  nOutputs=dspba_internal_get_channel_ports(gcb)  omode=Inherit via internal rule  otype=sfix(16)  scale=2^-15  rndmethod=Unbiased  factor=1  satmethod=Symmetric  shift_vec=[0 1 2 -1]  value=1  inPortNames=['v'; 'c'; '0'; '1'; '2'; '3'; '4'; '5'; '6'; '7'; '8'; '9'; 'A'; 'B'; 'D'; 'E'; 'F'; 'G'; 'H'; 'I'; 'J'; 'K'; 'L'; 'M'; 'N'; 'O'; 'P'; 'Q'; 'R'; 'S'; 'T'; 'U'; 'W'; 'X'; 'Y'; 'Z']  outPortNames=['v'; 'c'; '0'; '1'; '2'; '3'; '4'; '5'; '6'; '7'; '8'; '9'; 'A'; 'B'; 'D'; 'E'; 'F'; 'G'; 'H'; 'I'; 'J'; 'K'; 'L'; 'M'; 'N'; 'O'; 'P'; 'Q'; 'R'; 'S'; 'T'; 'U'; 'W'; 'X'; 'Y'; 'Z']  dspbaimage=dspba_prim.jpg  text=fprintf('Out%s', AdvDSPBChannelOutDisplay(latency));  style=Optimised  dataSignals=1  foldingEnabled=off  channels=1  sampleRate=200  packetBeginPresent=off  packetBeginEnabled=off  visibilities=dspba_ChannelOutVis(gcb)  latency=0  latencyCorrection=0  version=20141013
  ChannelOut1 : DSPBAPrim/ChannelOut  primtype=channelout  nInputs=dspba_internal_get_channel_ports(gcb)  nOutputs=dspba_internal_get_channel_ports(gcb)  omode=Inherit via internal rule  otype=sfix(16)  scale=2^-15  rndmethod=Unbiased  factor=1  satmethod=Symmetric  shift_vec=[0 1 2 -1]  value=1  inPortNames=['v'; 'c'; '0'; '1'; '2'; '3'; '4'; '5'; '6'; '7'; '8'; '9'; 'A'; 'B'; 'D'; 'E'; 'F'; 'G'; 'H'; 'I'; 'J'; 'K'; 'L'; 'M'; 'N'; 'O'; 'P'; 'Q'; 'R'; 'S'; 'T'; 'U'; 'W'; 'X'; 'Y'; 'Z']  outPortNames=['v'; 'c'; '0'; '1'; '2'; '3'; '4'; '5'; '6'; '7'; '8'; '9'; 'A'; 'B'; 'D'; 'E'; 'F'; 'G'; 'H'; 'I'; 'J'; 'K'; 'L'; 'M'; 'N'; 'O'; 'P'; 'Q'; 'R'; 'S'; 'T'; 'U'; 'W'; 'X'; 'Y'; 'Z']  dspbaimage=dspba_prim.jpg  text=fprintf('Out%s', AdvDSPBChannelOutDisplay(latency));  style=Optimised  dataSignals=1  foldingEnabled=off  channels=1  sampleRate=200  packetBeginPresent=off  packetBeginEnabled=off  visibilities=dspba_ChannelOutVis(gcb)  latency=0  latencyCorrection=0  version=20141013
  Const2 : DSPBAPrim/Const  primtype=const  nInputs=0  nOutputs=1  omode=boolean  otype=Boolean  scale=1  rndmethod=Unbiased  factor=1  satmethod=Symmetric  shift_vec=[0 1 2 -1]  value=0  inPortNames=['+'; '+';]  outPortNames=[' ']  dspbaimage=dspba_prim.jpg  text=fprintf('%s', num2str(value));  style=Optimised  visibilities=8 + 1024  floatPrecision=float32_m23  version=20120820
  Counter : DSPBAPrim/Counter  primtype=counter  nInputs=1  nOutputs=1  omode=Specify via dialog  otype=ufix(10)  scale=2^-0  rndmethod=Unbiased  factor=1  satmethod=Symmetric  shift_vec=[0 1 2 -1]  value=[0 memSize 1]  inPortNames=[' '; ' ';]  outPortNames=[' ']  dspbaimage=dspba_prim.jpg  text=fprintf('counter\n[%d %d %d]', value(1), value(2), value(3));  style=Optimised  visibilities=8 + 1024  version=20090407
  Counter1 : DSPBAPrim/Counter  primtype=counter  nInputs=1  nOutputs=1  omode=Specify via dialog  otype=ufix(10)  scale=2^-0  rndmethod=Unbiased  factor=1  satmethod=Symmetric  shift_vec=[0 1 2 -1]  value=[0 memSize 1]  inPortNames=[' '; ' ';]  outPortNames=[' ']  dspbaimage=dspba_prim.jpg  text=fprintf('counter\n[%d %d %d]', value(1), value(2), value(3));  style=Optimised  visibilities=8 + 1024  version=20090407
  DualMem : DSPBAPrim/DualMem  primtype=dualmem  nInputs=4  nOutputs=2  omode=Specify via dialog  otype=fixdt(1,wordLength)  scale=1  rndmethod=Unbiased  factor=1  satmethod=Symmetric  shift_vec=[0 1 2 -1]  value=memory_data  inPortNames=['d1'; 'a1'; 'w1'; 'a2']  outPortNames=['q1'; 'q2']  dspbaimage=dspba_prim.jpg  text=fprintf('dmem%s',AdvDSPBDMemDisplay(UseDontCare));  style=Optimised  visibilities=8 + 1024 + 2^17 + 2^18  UseDontCare=on  TwinWritePorts=off  version=20141001
  Mapper 1 : DSPBAPrim/Lut  primtype=lut  nInputs=1  nOutputs=1  omode=Specify via dialog  otype=sfix(2)  scale=1  rndmethod=Unbiased  factor=1  satmethod=Symmetric  shift_vec=[0 1 2 -1]  value=[-1 1]  inPortNames=[' '; ' ';]  outPortNames=[' ']  dspbaimage=dspba_prim.jpg  text=fprintf('LUT');  style=Optimised  visibilities=8 + 1024  floatPrecision=float32_m23  version=20090407
  Mode Meas : DSPBAPrim/Const  Commented=on  primtype=const  nInputs=0  nOutputs=1  omode=boolean  otype=ufix(1)  scale=1  rndmethod=Unbiased  factor=1  satmethod=Symmetric  shift_vec=[0 1 2 -1]  value=0  inPortNames=['+'; '+';]  outPortNames=[' ']  dspbaimage=dspba_prim.jpg  text=fprintf('%s', num2str(value));  style=Optimised  visibilities=8 + 1024  floatPrecision=float32_m23  version=20120820
  Not : DSPBAPrim/Not  primtype=not  nInputs=1  nOutputs=1  omode=Inherit via internal rule  otype=sfix(16)  scale=2^-15  rndmethod=Unbiased  factor=1  satmethod=Symmetric  shift_vec=[0 1 2 -1]  value=0  inPortNames=[' '; ' ';]  outPortNames=[' ']  dspbaimage=dspba_prim.jpg  text=fprintf('~');  style=Optimised  visibilities=8  version=20090407
  Not1 : DSPBAPrim/Not  primtype=not  nInputs=1  nOutputs=1  omode=Inherit via internal rule  otype=sfix(16)  scale=2^-15  rndmethod=Unbiased  factor=1  satmethod=Symmetric  shift_vec=[0 1 2 -1]  value=0  inPortNames=[' '; ' ';]  outPortNames=[' ']  dspbaimage=dspba_prim.jpg  text=fprintf('~');  style=Optimised  visibilities=8  version=20090407
  Not2 : DSPBAPrim/Not  Commented=on  primtype=not  nInputs=1  nOutputs=1  omode=Inherit via internal rule  otype=sfix(16)  scale=2^-15  rndmethod=Unbiased  factor=1  satmethod=Symmetric  shift_vec=[0 1 2 -1]  value=0  inPortNames=[' '; ' ';]  outPortNames=[' ']  dspbaimage=dspba_prim.jpg  text=fprintf('~');  style=Optimised  visibilities=8  version=20090407
  SRlatch : DSPBAControl/SRlatch  Commented=on
  SampleDelay2 : DSPBAPrim/SampleDelay  primtype=sampdelay  nInputs=1  nOutputs=1  omode=Inherit via internal rule  otype=sfix(16)  scale=2^-15  rndmethod=Unbiased  factor=1  satmethod=Symmetric  shift_vec=[0 1 2 -1]  value=1  inPortNames=[' '; ' ';]  outPortNames=[' ']  dspbaimage=dspba_prim.jpg  text=dpoly(1, eye(1,value+1), 'z')  style=Optimised  visibilities=8 + 1024 + 2^17 + 2^18  flexible=off  slackgroup=0  augmented=0  version=20090407  advOptions=[]
  Scope : Scope  NumInputPorts=3
  Scope1 : Scope  NumInputPorts=3
  Sequence : DSPBAPrim/Sequence  primtype=sequencer  nInputs=1  nOutputs=1  omode=Inherit via internal rule  otype=ufix(16)  scale=2^-0  rndmethod=Unbiased  factor=1  satmethod=Symmetric  shift_vec=[0 1 2 -1]  value=[0 1 sampleRate/dataRate]  inPortNames=[' '; ' ';]  outPortNames=[' ']  dspbaimage=dspba_prim.jpg  text=fprintf('seq\n[%d %d %d]', value(1), value(2), value(3));  style=Optimised  visibilities=1024  version=20090407
  Sequence1 : DSPBAPrim/Sequence  primtype=sequencer  nInputs=1  nOutputs=1  omode=Inherit via internal rule  otype=ufix(16)  scale=2^-0  rndmethod=Unbiased  factor=1  satmethod=Symmetric  shift_vec=[0 1 2 -1]  value=[35 1 sampleRate/dataRate]  inPortNames=[' '; ' ';]  outPortNames=[' ']  dspbaimage=dspba_prim.jpg  text=fprintf('seq\n[%d %d %d]', value(1), value(2), value(3));  style=Optimised  visibilities=1024  version=20090407
  Sequence2 : DSPBAPrim/Sequence  Commented=on  primtype=sequencer  nInputs=1  nOutputs=1  omode=Inherit via internal rule  otype=ufix(16)  scale=2^-0  rndmethod=Unbiased  factor=1  satmethod=Symmetric  shift_vec=[0 1 2 -1]  value=[0 1 pilot_size]  inPortNames=[' '; ' ';]  outPortNames=[' ']  dspbaimage=dspba_prim.jpg  text=fprintf('seq\n[%d %d %d]', value(1), value(2), value(3));  style=Optimised  visibilities=1024  version=20090407
  SynthesisInfo : DSPBAPrim/SynthesisInfo  primtype=synthinfo  nInputs=0  nOutputs=0  omode=Inherit via internal rule  otype=sfix(16)  scale=2^-15  rndmethod=Truncate  factor=1  satmethod=Symmetric  shift_vec=[0 1 2 -1]  value=99  inPortNames=[' '; ' ';]  outPortNames=[' ']  dspbaimage=dspba_prim_ctrl.jpg  text=fprintf('Style=%s', style);  style=Scheduled  visibilities=2^17+2^18+2^19+2^20  constraintInUse=off  constraintRelation=>  constraintLimit=2  bitAccurate=off  version=20150220
  m2 : Outport
  qv : Outport  Port=2
  qc : Outport  Port=3
  m1 : Outport  Port=4
  qv1 : Outport  Port=5
  qc1 : Outport  Port=6
  wires:
  ChannelIn/2 -> ChannelOut/2
  ChannelOut/2 -> qc/1
  dc/1 -> ChannelIn/2
  ChannelIn/1 -> Sequence/1
  Counter/1 -> DualMem/4
  ChannelOut/1 -> qv/1
  dv/1 -> ChannelIn/1
  ChannelOut/3 -> m2/1
  Const2/1 -> DualMem/1, DualMem/3
  Not/1 -> ChannelOut/1, Counter/1
  Sequence/1 -> Scope/3, Not/1
  Sequence1/1 -> Not1/1
  Mode Meas/1 -> SRlatch/2
  Sequence2/1 -> Not2/1
  trigger/1 -> ChannelIn1/1
  dc1/1 -> ChannelIn1/2
  ChannelOut1/3 -> m1/1
  ChannelOut1/1 -> qv1/1
  ChannelOut1/2 -> qc1/1
  ChannelIn1/1 -> And1/1, And3/2, Sequence1/1
  Not1/1 -> And1/2
  Counter1/1 -> DualMem/2
  ChannelIn1/2 -> ChannelOut1/2
  And1/1 -> ChannelOut1/1, SampleDelay2/1, And/1, Sequence2/1, And2/2, Scope1/3
  SampleDelay2/1 -> Counter1/1
  Not2/1 -> And2/1
  And2/1 -> SRlatch/1
  DualMem/1 -> And3/1, Scope1/2
  And3/1 -> ChannelOut1/3, Scope1/1
  Mapper 1/1 -> ChannelOut/3, Scope/1
  DualMem/2 -> Scope/2, Mapper 1/1
